simulink model "Lab4_2"  (R2024a)
settings: Solver=VariableStepAuto  StartTime=0.0  StopTime=25  MaxStep=0.1  RelTol=1e-3
settings Model: Creator=Pawel  LastModifiedBy=Pawel

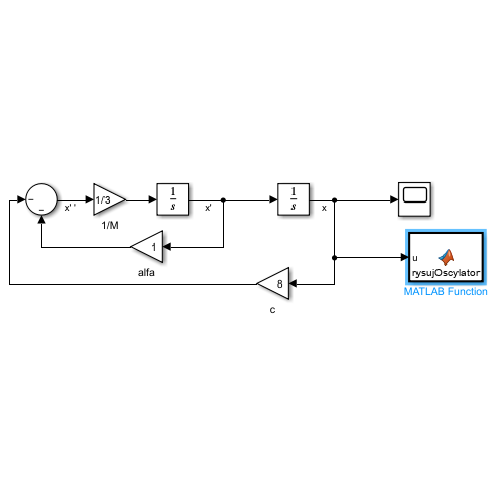
[thumbnail: Simulink's stored preview of the top-level diagram]
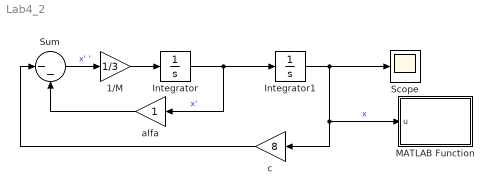
== system Lab4_2 ==
  1/M : Gain  Gain=1/3
  Integrator : Integrator  InitialCondition=2
  Integrator1 : Integrator  InitialCondition=1
  MATLAB Function : MATLAB Function  TreatAsAtomicUnit=on
  Scope : Scope
  Sum : Sum  Inputs=|--
  alfa : Gain
  c : Gain  Gain=8
  wires:
  Sum/1 -> 1/M/1  "x' '"
  Integrator/1 -> alfa/1, Integrator1/1  "x'"
  Integrator1/1 -> Scope/1, MATLAB Function/1(u), c/1  "x"
  1/M/1 -> Integrator/1
  alfa/1 -> Sum/2
  c/1 -> Sum/1

== matlab function Lab4_2/MATLAB Function ==
  data: u input
function rysujOscylator(u)

position = u(1);

cla
hold on;
fill([-2,-2,2,2], [2,1.9,1.9,2], 'b')
plot(0, position, 'rs', 'MarkerSize', 60, 'MarkerFaceColor', 'r')
xlim([-2 2])
ylim([-2 2])

springWidth = 0.05; % Szerokość sprężyny
springColor = [0.8 0.8 0.8]; % Kolor sprężyny
springY = linspace(1.95, position, 11); % Początek od sufitu
% Rysowanie sprężyny jako wielu segmentów linii
for i = 1:10
    springSegmentY = linspace(springY(i), springY(i+1), 20);
    springSegmentX = springWidth * sin(linspace(0, pi, 20));
    plot(springSegmentX, springSegmentY, 'Color', springColor, 'LineWidth', 1.5);
end

hold off
axis off

drawnow
